simulink subsystem "petite_cana_complexeV2"  (R2024a)
settings: Solver=VariableStepAuto  StartTime=0.0  StopTime=10.0  RelTol=1e-3
undefined symbols (not defined in the file): Connection1, Connection10, Connection11, Connection12, Connection2, Connection3, Connection4, Connection5, Connection6, Connection7, Connection8, Connection9, longueur_cana, pipeline, X, Y, Z
libraries: sm_lib x27, nesl_utility x12
settings Model: Creator=vincp  LastModifiedBy=VincentPERRET

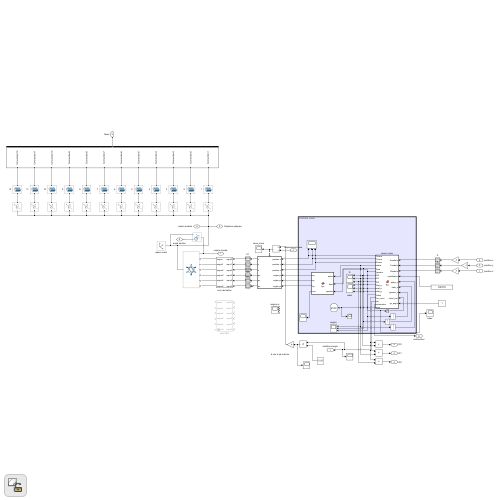
[thumbnail: Simulink's stored preview of the top-level diagram]
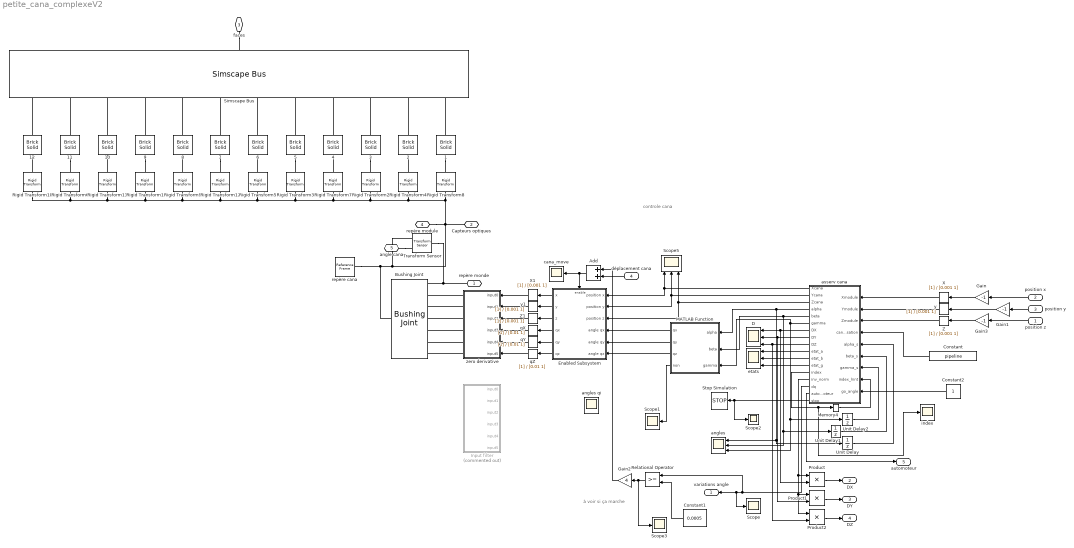
== system petite_cana_complexeV2 ==
  note: à voir si ça marche
  note: controle cana
  position z : Inport
  position x : Inport  Port=2
  position y : Inport  Port=3
  déplacement cana : Inport  Port=4
  " 1" : sm_lib/Body Elements/Brick Solid  BrickDimensions=dim_cana  BrickDimensionsUnits=m  ExportEntireGeometry=on  InertiaType=CalculateFromGeometry  BasedOnType=Mass  Density=1000  DensityUnits=kg/m^3  Mass=0  MassUnits=kg  CenterOfMass=[0 0 0]  CenterOfMassUnits=m  MomentsOfInertia=[1 1 1]  MomentsOfInertiaUnits=kg*m^2  ProductsOfInertia=[0 0 0]  ProductsOfInertiaUnits=kg*m^2  GraphicType=FromGeometry  MarkerShape=Sphere  MarkerSize=10  GraphicVisPropType=SimpleVisualProperties  GraphicDiffuseColor=[0.0 0.0 0.0]  GraphicOpacity=0.3  GraphicSpecularColor=[0.5 0.5 0.5 1.0]  GraphicAmbientColor=[0.15 0.15 0.15 1.0]  GraphicEmissiveColor=[0.0 0.0 0.0 1.0]  GraphicShininess=75  DoExposeReferenceFrame=on  SerializedFrames=<Frames/>
  " 2" : sm_lib/Body Elements/Brick Solid  BrickDimensions=dim_cana  BrickDimensionsUnits=m  ExportEntireGeometry=on  InertiaType=CalculateFromGeometry  BasedOnType=Mass  Density=1000  DensityUnits=kg/m^3  Mass=0  MassUnits=kg  CenterOfMass=[0 0 0]  CenterOfMassUnits=m  MomentsOfInertia=[1 1 1]  MomentsOfInertiaUnits=kg*m^2  ProductsOfInertia=[0 0 0]  ProductsOfInertiaUnits=kg*m^2  GraphicType=FromGeometry  MarkerShape=Sphere  MarkerSize=10  GraphicVisPropType=SimpleVisualProperties  GraphicDiffuseColor=[0.0 0.0 0.0]  GraphicOpacity=0.3  GraphicSpecularColor=[0.5 0.5 0.5 1.0]  GraphicAmbientColor=[0.15 0.15 0.15 1.0]  GraphicEmissiveColor=[0.0 0.0 0.0 1.0]  GraphicShininess=75  DoExposeReferenceFrame=on  SerializedFrames=<Frames/>
  {3,8,10,12} (4 alike) : sm_lib/Body Elements/Brick Solid  BrickDimensions=dim_cana  BrickDimensionsUnits=m  ExportEntireGeometry=on  InertiaType=CalculateFromGeometry  BasedOnType=Mass  Density=0  DensityUnits=kg/m^3  Mass=0  MassUnits=kg  CenterOfMass=[0 0 0]  CenterOfMassUnits=m  MomentsOfInertia=[1 1 1]  MomentsOfInertiaUnits=kg*m^2  ProductsOfInertia=[0 0 0]  ProductsOfInertiaUnits=kg*m^2  GraphicType=FromGeometry  MarkerShape=Sphere  MarkerSize=10  GraphicVisPropType=SimpleVisualProperties  GraphicDiffuseColor=[0.0 0.0 0.0]  GraphicOpacity=0.3  GraphicSpecularColor=[0.5 0.5 0.5 1.0]  GraphicAmbientColor=[0.15 0.15 0.15 1.0]  GraphicEmissiveColor=[0.0 0.0 0.0 1.0]  GraphicShininess=75  DoExposeReferenceFrame=on  SerializedFrames=<Frames/>
  {4..7,9,11} (6 alike) : sm_lib/Body Elements/Brick Solid  BrickDimensions=dim_cana  BrickDimensionsUnits=m  ExportEntireGeometry=on  InertiaType=CalculateFromGeometry  BasedOnType=Mass  Density=1000  DensityUnits=kg/m^3  Mass=0  MassUnits=kg  CenterOfMass=[0 0 0]  CenterOfMassUnits=m  MomentsOfInertia=[1 1 1]  MomentsOfInertiaUnits=kg*m^2  ProductsOfInertia=[0 0 0]  ProductsOfInertiaUnits=kg*m^2  GraphicType=FromGeometry  MarkerShape=Sphere  MarkerSize=10  GraphicVisPropType=SimpleVisualProperties  GraphicDiffuseColor=[0.0 0.0 0.0]  GraphicOpacity=0.3  GraphicSpecularColor=[0.5 0.5 0.5 1.0]  GraphicAmbientColor=[0.15 0.15 0.15 1.0]  GraphicEmissiveColor=[0.0 0.0 0.0 1.0]  GraphicShininess=75  DoExposeReferenceFrame=on  SerializedFrames=<Frames/>
  Add : Sum
  Bushing Joint : sm_lib/Joints/Bushing Joint  JointMode=Normal  CompositeWrenchDir=FollowerOnBase  CompositeWrenchFrame=BaseFrame  SenseConstraintForce=off  SenseConstraintTorque=off  SenseTotalForce=off  SenseTotalTorque=off  PxPositionTargetSpecify=off  PxPositionTargetPriority=High  PxPositionTargetValue=0  PxPositionTargetValueUnits=m  PxVelocityTargetSpecify=off  PxVelocityTargetPriority=High  PxVelocityTargetValue=0  PxVelocityTargetValueUnits=m/s  PxEquilibriumPosition=0  PxEquilibriumPositionUnits=m  PxSpringStiffness=0  PxSpringStiffnessUnits=N/m  PxDampingCoefficient=0  PxDampingCoefficientUnits=N/(m/s)  PxLowerLimitSpecify=off  PxLowerLimitBound=-1  PxLowerLimitBoundUnits=m  PxLowerLimitStiffness=1e6  PxLowerLimitStiffnessUnits=N/m  PxLowerLimitDamping=1e3  PxLowerLimitDampingUnits=N/(m/s)  PxLowerLimitTransitionRegionWidth=1e-4  PxLowerLimitTransitionRegionWidthUnits=m  PxUpperLimitSpecify=off  PxUpperLimitBound=1  PxUpperLimitBoundUnits=m  PxUpperLimitStiffness=1e6  PxUpperLimitStiffnessUnits=N/m  PxUpperLimitDamping=1e3  PxUpperLimitDampingUnits=N/(m/s)  PxUpperLimitTransitionRegionWidth=1e-4  PxUpperLimitTransitionRegionWidthUnits=m  PxTorqueActuationMode=ComputedTorque  PxMotionActuationMode=InputMotion  PxSensePosition=off  PxSenseVelocity=off  PxSenseAcceleration=off  PxSenseTorqueForce=off  PxSenseLowerLimitTorqueForce=off  PxSenseUpperLimitTorqueForce=off  PyPositionTargetSpecify=off  PyPositionTargetPriority=High  PyPositionTargetValue=0  PyPositionTargetValueUnits=m  PyVelocityTargetSpecify=off  PyVelocityTargetPriority=High  PyVelocityTargetValue=0  PyVelocityTargetValueUnits=m/s  PyEquilibriumPosition=0  PyEquilibriumPositionUnits=m  PySpringStiffness=0  PySpringStiffnessUnits=N/m  PyDampingCoefficient=0  PyDampingCoefficientUnits=N/(m/s)  PyLowerLimitSpecify=off  PyLowerLimitBound=-1  PyLowerLimitBoundUnits=m  PyLowerLimitStiffness=1e6  PyLowerLimitStiffnessUnits=N/m  PyLowerLimitDamping=1e3  PyLowerLimitDampingUnits=N/(m/s)  PyLowerLimitTransitionRegionWidth=1e-4  PyLowerLimitTransitionRegionWidthUnits=m  PyUpperLimitSpecify=off  PyUpperLimitBound=1  PyUpperLimitBoundUnits=m  PyUpperLimitStiffness=1e6  PyUpperLimitStiffnessUnits=N/m  PyUpperLimitDamping=1e3  PyUpperLimitDampingUnits=N/(m/s)  PyUpperLimitTransitionRegionWidth=1e-4  PyUpperLimitTransitionRegionWidthUnits=m  PyTorqueActuationMode=ComputedTorque  PyMotionActuationMode=InputMotion  PySensePosition=off  PySenseVelocity=off  PySenseAcceleration=off  PySenseTorqueForce=off  PySenseLowerLimitTorqueForce=off  PySenseUpperLimitTorqueForce=off  PzPositionTargetSpecify=off  PzPositionTargetPriority=High  PzPositionTargetValue=0  PzPositionTargetValueUnits=m  PzVelocityTargetSpecify=off  PzVelocityTargetPriority=High  PzVelocityTargetValue=0  PzVelocityTargetValueUnits=m/s  PzEquilibriumPosition=0  PzEquilibriumPositionUnits=m  PzSpringStiffness=0  PzSpringStiffnessUnits=N/m  PzDampingCoefficient=0  PzDampingCoefficientUnits=N/(m/s)  PzLowerLimitSpecify=off  PzLowerLimitBound=-1  PzLowerLimitBoundUnits=m  PzLowerLimitStiffness=1e6  PzLowerLimitStiffnessUnits=N/m  PzLowerLimitDamping=1e3  PzLowerLimitDampingUnits=N/(m/s)  PzLowerLimitTransitionRegionWidth=1e-4  PzLowerLimitTransitionRegionWidthUnits=m  PzUpperLimitSpecify=off  PzUpperLimitBound=1  PzUpperLimitBoundUnits=m  PzUpperLimitStiffness=1e6  PzUpperLimitStiffnessUnits=N/m  PzUpperLimitDamping=1e3  PzUpperLimitDampingUnits=N/(m/s)  PzUpperLimitTransitionRegionWidth=1e-4  PzUpperLimitTransitionRegionWidthUnits=m  PzTorqueActuationMode=ComputedTorque  PzMotionActuationMode=InputMotion  PzSensePosition=off  PzSenseVelocity=off  PzSenseAcceleration=off  PzSenseTorqueForce=off  PzSenseLowerLimitTorqueForce=off  PzSenseUpperLimitTorqueForce=off  RxPositionTargetSpecify=off  RxPositionTargetPriority=High  RxPositionTargetValue=0  RxPositionTargetValueUnits=deg  RxVelocityTargetSpecify=off  RxVelocityTargetPriority=High  RxVelocityTargetValue=0  RxVelocityTargetValueUnits=deg/s  RxEquilibriumPosition=0  RxEquilibriumPositionUnits=deg  RxSpringStiffness=0  RxSpringStiffnessUnits=N*m/deg  RxDampingCoefficient=0  RxDampingCoefficientUnits=N*m/(deg/s)  RxLowerLimitSpecify=off  RxLowerLimitBound=-90  RxLowerLimitBoundUnits=deg  RxLowerLimitStiffness=1e4  RxLowerLimitStiffnessUnits=N*m/deg  RxLowerLimitDamping=10  RxLowerLimitDampingUnits=N*m/(deg/s)  RxLowerLimitTransitionRegionWidth=0.1  RxLowerLimitTransitionRegionWidthUnits=deg  RxUpperLimitSpecify=off  RxUpperLimitBound=90  RxUpperLimitBoundUnits=deg  RxUpperLimitStiffness=1e4  RxUpperLimitStiffnessUnits=N*m/deg  RxUpperLimitDamping=10  RxUpperLimitDampingUnits=N*m/(deg/s)  RxUpperLimitTransitionRegionWidth=0.1  RxUpperLimitTransitionRegionWidthUnits=deg  RxTorqueActuationMode=ComputedTorque  RxMotionActuationMode=InputMotion  RxSensePosition=off  RxSenseVelocity=off  RxSenseAcceleration=off  RxSenseTorqueForce=off  RxSenseLowerLimitTorqueForce=off  RxSenseUpperLimitTorqueForce=off  RyPositionTargetSpecify=off  RyPositionTargetPriority=High  RyPositionTargetValue=0  RyPositionTargetValueUnits=deg  RyVelocityTargetSpecify=off  RyVelocityTargetPriority=High  RyVelocityTargetValue=0  RyVelocityTargetValueUnits=deg/s  RyEquilibriumPosition=0  RyEquilibriumPositionUnits=deg  RySpringStiffness=0  RySpringStiffnessUnits=N*m/deg  RyDampingCoefficient=0  RyDampingCoefficientUnits=N*m/(deg/s)  RyLowerLimitSpecify=off  RyLowerLimitBound=-90  RyLowerLimitBoundUnits=deg  RyLowerLimitStiffness=1e4  RyLowerLimitStiffnessUnits=N*m/deg  RyLowerLimitDamping=10  RyLowerLimitDampingUnits=N*m/(deg/s)  RyLowerLimitTransitionRegionWidth=0.1  RyLowerLimitTransitionRegionWidthUnits=deg  RyUpperLimitSpecify=off  RyUpperLimitBound=90  RyUpperLimitBoundUnits=deg  RyUpperLimitStiffness=1e4  RyUpperLimitStiffnessUnits=N*m/deg  RyUpperLimitDamping=10  RyUpperLimitDampingUnits=N*m/(deg/s)  RyUpperLimitTransitionRegionWidth=0.1  RyUpperLimitTransitionRegionWidthUnits=deg  RyTorqueActuationMode=ComputedTorque  RyMotionActuationMode=InputMotion  RySensePosition=off  RySenseVelocity=off  RySenseAcceleration=off  RySenseTorqueForce=off  RySenseLowerLimitTorqueForce=off  RySenseUpperLimitTorqueForce=off  RzPositionTargetSpecify=off  RzPositionTargetPriority=High  RzPositionTargetValue=0  RzPositionTargetValueUnits=deg  RzVelocityTargetSpecify=off  RzVelocityTargetPriority=High  RzVelocityTargetValue=0  RzVelocityTargetValueUnits=deg/s  RzEquilibriumPosition=0  RzEquilibriumPositionUnits=deg  RzSpringStiffness=0  RzSpringStiffnessUnits=N*m/deg  RzDampingCoefficient=0  RzDampingCoefficientUnits=N*m/(deg/s)  RzLowerLimitSpecify=off  RzLowerLimitBound=-90  RzLowerLimitBoundUnits=deg  RzLowerLimitStiffness=1e4  RzLowerLimitStiffnessUnits=N*m/deg  RzLowerLimitDamping=10  RzLowerLimitDampingUnits=N*m/(deg/s)  RzLowerLimitTransitionRegionWidth=0.1  RzLowerLimitTransitionRegionWidthUnits=deg  RzUpperLimitSpecify=off  RzUpperLimitBound=90  RzUpperLimitBoundUnits=deg  RzUpperLimitStiffness=1e4  RzUpperLimitStiffnessUnits=N*m/deg  RzUpperLimitDamping=10  RzUpperLimitDampingUnits=N*m/(deg/s)  RzUpperLimitTransitionRegionWidth=0.1  RzUpperLimitTransitionRegionWidthUnits=deg  RzTorqueActuationMode=ComputedTorque  RzMotionActuationMode=InputMotion  RzSensePosition=off  RzSenseVelocity=off  RzSenseAcceleration=off  RzSenseTorqueForce=off  RzSenseLowerLimitTorqueForce=off  RzSenseUpperLimitTorqueForce=off
  Constant : Constant  Value=pipeline
  Constant1 : Constant  Value=0.0005
  Constant2 : Constant
  D : Scope  NumInputPorts=3
  Enabled Subsystem : Subsystem  TreatAsAtomicUnit=on
  Gain : Gain  Gain=-1
  Gain1 : Gain  Gain=-1
  Gain2 : Gain  Gain=4
  Gain3 : Gain  Gain=-1
  Input filter : Subsystem  Commented=on
  MATLAB Function : MATLAB Function  TreatAsAtomicUnit=on
  Memory4 : Memory  InitialCondition=1  InheritSampleTime=on  LinearizeAsDelay=on
  Product : Product
  Product1 : Product
  Product2 : Product
  Relational Operator : RelationalOperator  OutDataTypeStr=boolean  RndMeth=Simplest  InputSameDT=off
  Rigid Transform1 : sm_lib/Frames and Transforms/Rigid Transform  RotationMethod=StandardAxis  FollAlignAxisA=+X  BaseAlignAxisA=+Y  FollAlignAxisB=+Y  BaseAlignAxisB=+Z  RotationStandardAxis=+Z  RotationAngle=-60  RotationAngleUnits=deg  RotationArbitraryAxis=[0 0 1]  RotationSequenceAxes=FollowerAxes  RotationSequence=XYX  RotationSequenceAngles=[0 0 0]  RotationSequenceAnglesUnits=deg  RotationMatrix=[1 0 0; 0 1 0; 0 0 1]  Quaternion=[1 0 0 0]  TranslationMethod=Cartesian  TranslationCartesianOffset=[-125*sin(4*pi/12) -125*cos(4*pi/12) longueur_cana*500-150]  TranslationCartesianOffsetUnits=mm  TranslationStandardAxis=+Y  TranslationStandardOffset=125  TranslationStandardOffsetUnits=mm  TranslationROffset=0  TranslationROffsetUnits=m  TranslationThetaOffset=0  TranslationThetaOffsetUnits=deg  TranslationZOffset=0  TranslationZOffsetUnits=m
  Rigid Transform10 : sm_lib/Frames and Transforms/Rigid Transform  RotationMethod=StandardAxis  FollAlignAxisA=+X  BaseAlignAxisA=+Y  FollAlignAxisB=+Y  BaseAlignAxisB=+Z  RotationStandardAxis=+Z  RotationAngle=90  RotationAngleUnits=deg  RotationArbitraryAxis=[0 0 1]  RotationSequenceAxes=FollowerAxes  RotationSequence=XYX  RotationSequenceAngles=[0 0 0]  RotationSequenceAnglesUnits=deg  RotationMatrix=[1 0 0; 0 1 0; 0 0 1]  Quaternion=[1 0 0 0]  TranslationMethod=Cartesian  TranslationCartesianOffset=[-125 0 longueur_cana*500-150]  TranslationCartesianOffsetUnits=mm  TranslationStandardAxis=+Y  TranslationStandardOffset=125  TranslationStandardOffsetUnits=mm  TranslationROffset=0  TranslationROffsetUnits=m  TranslationThetaOffset=0  TranslationThetaOffsetUnits=deg  TranslationZOffset=0  TranslationZOffsetUnits=m
  Rigid Transform11 : sm_lib/Frames and Transforms/Rigid Transform  RotationMethod=StandardAxis  FollAlignAxisA=+X  BaseAlignAxisA=+Y  FollAlignAxisB=+Y  BaseAlignAxisB=+Z  RotationStandardAxis=+Z  RotationAngle=30  RotationAngleUnits=deg  RotationArbitraryAxis=[0 0 1]  RotationSequenceAxes=FollowerAxes  RotationSequence=XYX  RotationSequenceAngles=[0 0 0]  RotationSequenceAnglesUnits=deg  RotationMatrix=[1 0 0; 0 1 0; 0 0 1]  Quaternion=[1 0 0 0]  TranslationMethod=Cartesian  TranslationCartesianOffset=[125*sin(14*pi/12) -125*cos(14*pi/12) longueur_cana*500-150]  TranslationCartesianOffsetUnits=mm  TranslationStandardAxis=+Y  TranslationStandardOffset=125  TranslationStandardOffsetUnits=mm  TranslationROffset=0  TranslationROffsetUnits=m  TranslationThetaOffset=0  TranslationThetaOffsetUnits=deg  TranslationZOffset=0  TranslationZOffsetUnits=m
  Rigid Transform12 : sm_lib/Frames and Transforms/Rigid Transform  RotationMethod=StandardAxis  FollAlignAxisA=+X  BaseAlignAxisA=+Y  FollAlignAxisB=+Y  BaseAlignAxisB=+Z  RotationStandardAxis=+Z  RotationAngle=-30  RotationAngleUnits=deg  RotationArbitraryAxis=[0 0 1]  RotationSequenceAxes=FollowerAxes  RotationSequence=XYX  RotationSequenceAngles=[0 0 0]  RotationSequenceAnglesUnits=deg  RotationMatrix=[1 0 0; 0 1 0; 0 0 1]  Quaternion=[1 0 0 0]  TranslationMethod=Cartesian  TranslationCartesianOffset=[-125*sin(2*pi/12) -125*cos(2*pi/12) longueur_cana*500-150]  TranslationCartesianOffsetUnits=mm  TranslationStandardAxis=+Y  TranslationStandardOffset=125  TranslationStandardOffsetUnits=mm  TranslationROffset=0  TranslationROffsetUnits=m  TranslationThetaOffset=0  TranslationThetaOffsetUnits=deg  TranslationZOffset=0  TranslationZOffsetUnits=m
  Rigid Transform2 : sm_lib/Frames and Transforms/Rigid Transform  RotationMethod=StandardAxis  FollAlignAxisA=+X  BaseAlignAxisA=+Y  FollAlignAxisB=+Y  BaseAlignAxisB=+Z  RotationStandardAxis=+Z  RotationAngle=60  RotationAngleUnits=deg  RotationArbitraryAxis=[0 0 1]  RotationSequenceAxes=FollowerAxes  RotationSequence=XYX  RotationSequenceAngles=[0 0 0]  RotationSequenceAnglesUnits=deg  RotationMatrix=[1 0 0; 0 1 0; 0 0 1]  Quaternion=[1 0 0 0]  TranslationMethod=Cartesian  TranslationCartesianOffset=[125*sin(4*pi/12) -125*cos(4*pi/12) longueur_cana*500-150]  TranslationCartesianOffsetUnits=mm  TranslationStandardAxis=+Y  TranslationStandardOffset=125  TranslationStandardOffsetUnits=mm  TranslationROffset=0  TranslationROffsetUnits=m  TranslationThetaOffset=0  TranslationThetaOffsetUnits=deg  TranslationZOffset=0  TranslationZOffsetUnits=m
  Rigid Transform3 : sm_lib/Frames and Transforms/Rigid Transform  RotationMethod=StandardAxis  FollAlignAxisA=+X  BaseAlignAxisA=+Y  FollAlignAxisB=+Y  BaseAlignAxisB=+Z  RotationStandardAxis=+Z  RotationAngle=120  RotationAngleUnits=deg  RotationArbitraryAxis=[0 0 1]  RotationSequenceAxes=FollowerAxes  RotationSequence=XYX  RotationSequenceAngles=[0 0 0]  RotationSequenceAnglesUnits=deg  RotationMatrix=[1 0 0; 0 1 0; 0 0 1]  Quaternion=[1 0 0 0]  TranslationMethod=Cartesian  TranslationCartesianOffset=[125*sin(8*pi/12) -125*cos(8*pi/12) longueur_cana*500-150]  TranslationCartesianOffsetUnits=mm  TranslationStandardAxis=+Y  TranslationStandardOffset=125  TranslationStandardOffsetUnits=mm  TranslationROffset=0  TranslationROffsetUnits=m  TranslationThetaOffset=0  TranslationThetaOffsetUnits=deg  TranslationZOffset=0  TranslationZOffsetUnits=m
  Rigid Transform4 : sm_lib/Frames and Transforms/Rigid Transform  RotationMethod=StandardAxis  FollAlignAxisA=+X  BaseAlignAxisA=+Y  FollAlignAxisB=+Y  BaseAlignAxisB=+Z  RotationStandardAxis=+Z  RotationAngle=30  RotationAngleUnits=deg  RotationArbitraryAxis=[0 0 1]  RotationSequenceAxes=FollowerAxes  RotationSequence=XYX  RotationSequenceAngles=[0 0 0]  RotationSequenceAnglesUnits=deg  RotationMatrix=[1 0 0; 0 1 0; 0 0 1]  Quaternion=[1 0 0 0]  TranslationMethod=Cartesian  TranslationCartesianOffset=[125*sin(2*pi/12) -125*cos(2*pi/12) longueur_cana*500-150]  TranslationCartesianOffsetUnits=mm  TranslationStandardAxis=+Y  TranslationStandardOffset=125  TranslationStandardOffsetUnits=mm  TranslationROffset=0  TranslationROffsetUnits=m  TranslationThetaOffset=0  TranslationThetaOffsetUnits=deg  TranslationZOffset=0  TranslationZOffsetUnits=m
  Rigid Transform5 : sm_lib/Frames and Transforms/Rigid Transform  RotationMethod=StandardAxis  FollAlignAxisA=+X  BaseAlignAxisA=+Y  FollAlignAxisB=+Y  BaseAlignAxisB=+Z  RotationStandardAxis=+Z  RotationAngle=150  RotationAngleUnits=deg  RotationArbitraryAxis=[0 0 1]  RotationSequenceAxes=FollowerAxes  RotationSequence=XYX  RotationSequenceAngles=[0 0 0]  RotationSequenceAnglesUnits=deg  RotationMatrix=[1 0 0; 0 1 0; 0 0 1]  Quaternion=[1 0 0 0]  TranslationMethod=Cartesian  TranslationCartesianOffset=[125*sin(10*pi/12) -125*cos(10*pi/12) longueur_cana*500-150]  TranslationCartesianOffsetUnits=mm  TranslationStandardAxis=+Y  TranslationStandardOffset=125  TranslationStandardOffsetUnits=mm  TranslationROffset=0  TranslationROffsetUnits=m  TranslationThetaOffset=0  TranslationThetaOffsetUnits=deg  TranslationZOffset=0  TranslationZOffsetUnits=m
  Rigid Transform6 : sm_lib/Frames and Transforms/Rigid Transform  RotationMethod=StandardAxis  FollAlignAxisA=+X  BaseAlignAxisA=+Y  FollAlignAxisB=+Y  BaseAlignAxisB=+Z  RotationStandardAxis=+Z  RotationAngle=60  RotationAngleUnits=deg  RotationArbitraryAxis=[0 0 1]  RotationSequenceAxes=FollowerAxes  RotationSequence=XYX  RotationSequenceAngles=[0 0 0]  RotationSequenceAnglesUnits=deg  RotationMatrix=[1 0 0; 0 1 0; 0 0 1]  Quaternion=[1 0 0 0]  TranslationMethod=Cartesian  TranslationCartesianOffset=[-125*cos(pi/6) 125*sin(pi/6) longueur_cana*500-150]  TranslationCartesianOffsetUnits=mm  TranslationStandardAxis=+Y  TranslationStandardOffset=125  TranslationStandardOffsetUnits=mm  TranslationROffset=0  TranslationROffsetUnits=m  TranslationThetaOffset=0  TranslationThetaOffsetUnits=deg  TranslationZOffset=0  TranslationZOffsetUnits=m
  Rigid Transform7 : sm_lib/Frames and Transforms/Rigid Transform  RotationMethod=StandardAxis  FollAlignAxisA=+X  BaseAlignAxisA=+Y  FollAlignAxisB=+Y  BaseAlignAxisB=+Z  RotationStandardAxis=+Z  RotationAngle=90  RotationAngleUnits=deg  RotationArbitraryAxis=[0 0 1]  RotationSequenceAxes=FollowerAxes  RotationSequence=XYX  RotationSequenceAngles=[0 0 0]  RotationSequenceAnglesUnits=deg  RotationMatrix=[1 0 0; 0 1 0; 0 0 1]  Quaternion=[1 0 0 0]  TranslationMethod=Cartesian  TranslationCartesianOffset=[125 0 longueur_cana*500-150]  TranslationCartesianOffsetUnits=mm  TranslationStandardAxis=+Y  TranslationStandardOffset=125  TranslationStandardOffsetUnits=mm  TranslationROffset=0  TranslationROffsetUnits=m  TranslationThetaOffset=0  TranslationThetaOffsetUnits=deg  TranslationZOffset=0  TranslationZOffsetUnits=m
  Rigid Transform8 : sm_lib/Frames and Transforms/Rigid Transform  RotationMethod=StandardAxis  FollAlignAxisA=+X  BaseAlignAxisA=+Y  FollAlignAxisB=+Y  BaseAlignAxisB=+Z  RotationStandardAxis=+Z  RotationAngle=0  RotationAngleUnits=deg  RotationArbitraryAxis=[0 0 1]  RotationSequenceAxes=FollowerAxes  RotationSequence=XYX  RotationSequenceAngles=[0 0 0]  RotationSequenceAnglesUnits=deg  RotationMatrix=[1 0 0; 0 1 0; 0 0 1]  Quaternion=[1 0 0 0]  TranslationMethod=Cartesian  TranslationCartesianOffset=[0 -125 longueur_cana*500-150]  TranslationCartesianOffsetUnits=mm  TranslationStandardAxis=+Y  TranslationStandardOffset=125  TranslationStandardOffsetUnits=mm  TranslationROffset=0  TranslationROffsetUnits=m  TranslationThetaOffset=0  TranslationThetaOffsetUnits=deg  TranslationZOffset=0  TranslationZOffsetUnits=m
  Rigid Transform9 : sm_lib/Frames and Transforms/Rigid Transform  RotationMethod=StandardAxis  FollAlignAxisA=+X  BaseAlignAxisA=+Y  FollAlignAxisB=+Y  BaseAlignAxisB=+Z  RotationStandardAxis=+Z  RotationAngle=0  RotationAngleUnits=deg  RotationArbitraryAxis=[0 0 1]  RotationSequenceAxes=FollowerAxes  RotationSequence=XYX  RotationSequenceAngles=[0 0 0]  RotationSequenceAnglesUnits=deg  RotationMatrix=[1 0 0; 0 1 0; 0 0 1]  Quaternion=[1 0 0 0]  TranslationMethod=Cartesian  TranslationCartesianOffset=[0 125 longueur_cana*500-150]  TranslationCartesianOffsetUnits=mm  TranslationStandardAxis=+Y  TranslationStandardOffset=125  TranslationStandardOffsetUnits=mm  TranslationROffset=0  TranslationROffsetUnits=m  TranslationThetaOffset=0  TranslationThetaOffsetUnits=deg  TranslationZOffset=0  TranslationZOffsetUnits=m
  Scope{,1..3} (4 alike) : Scope
  Scope5 : Scope  NumInputPorts=3
  Simscape Bus : SimscapeBus  HierarchyStrings=Connection12;Connection11;Connection10;Connection9;Connection8;Connection7;Connection6;Connection5;Connection4;Connection3;Connection2;Connection1
  Stop Simulation : Stop
  Transform Sensor : sm_lib/Frames and Transforms/Transform Sensor  MeasurementFrame=World  RotationSequence=XYX  SenseAngle=on  SenseAxis=off  SenseQ=off  SenseR=off  SenseRotationSequence=off  SenseOmegaX=off  SenseOmegaY=off  SenseOmegaZ=off  SenseOmega=off  SenseQDot=off  SenseRDot=off  SenseRotationSequenceDot=off  SenseAlphaX=off  SenseAlphaY=off  SenseAlphaZ=off  SenseAlpha=off  SenseQDDot=off  SenseRDDot=off  SenseX=off  SenseY=off  SenseZ=off  SenseXYZ=off  SenseRad=off  SenseAzim=off  SenseDist=off  SenseInc=off  SenseXDot=off  SenseYDot=off  SenseZDot=off  SenseXYZDot=off  SenseRadDot=off  SenseAzimDot=off  SenseDistDot=off  SenseIncDot=off  SenseXDDot=off  SenseYDDot=off  SenseZDDot=off  SenseXYZDDot=off  SenseRadDDot=off  SenseAzimDDot=off  SenseDistDDot=off  SenseIncDDot=off
  Unit Delay : UnitDelay  SampleTime=-1  HasFrameUpgradeWarning=on
  Unit Delay1 : UnitDelay  SampleTime=-1  HasFrameUpgradeWarning=on
  Unit Delay2 : UnitDelay  SampleTime=-1  HasFrameUpgradeWarning=on
  X : TransferFcn  Denominator=[0.001 1]
  X1 : TransferFcn  Denominator=[0.001 1]
  Z : TransferFcn  Denominator=[0.001 1]
  Z1 : TransferFcn  Denominator=[0.001 1]
  angles : Scope  NumInputPorts=3
  angles qi : Scope  NumInputPorts=3
  asserv cana : MATLAB Function  TreatAsAtomicUnit=on
  cana_move : Scope
  etats : Scope  NumInputPorts=3
  index : Scope
  qX : TransferFcn  Denominator=[0.01 1]
  qY : TransferFcn  Denominator=[0.01 1]
  qZ : TransferFcn  Denominator=[0.01 1]
  repère cana : sm_lib/Frames and Transforms/Reference Frame
  y : TransferFcn  Denominator=[0.001 1]
  y1 : TransferFcn  Denominator=[0.001 1]
  zero derivative : Subsystem
  repère monde : PMIOPort  Side=Right
  Capteurs optiques : PMIOPort  Port=2  Side=Left
  faces : PMIOPort  Port=3  Side=Left
  repère module : PMIOPort  Port=4  Side=Left
  angle cana : PMIOPort  Port=5  Side=Left
  variations angle : Outport
  DX : Outport  Port=2
  DY : Outport  Port=3
  DZ : Outport  Port=4
  automoteur : Outport  Port=5
  wires:
  position y/1 -> Gain1/1
  position z/1 -> Gain3/1
  Gain1/1 -> y/1
  Gain3/1 -> Z/1
  Gain/1 -> X/1
  asserv cana/1(Xcana) -> Scope5/1, Enabled Subsystem/1(position x)
  asserv cana/2(Ycana) -> Scope5/2, Enabled Subsystem/2(position y)
  asserv cana/3(Zcana) -> Scope5/3, Enabled Subsystem/3(position z)
  Z/1 -> asserv cana/3(Zmodule)
  asserv cana/7(DX) -> D/1, Product/2
  asserv cana/9(DZ) -> D/3, Product2/2
  Constant/1 -> asserv cana/4(canalisation)
  asserv cana/12(etat_g) -> etats/3
  Constant2/1 -> asserv cana/9(go_angle)
  Memory4/1 -> asserv cana/8(index_hint)
  asserv cana/13(index) -> Memory4/1, index/1
  Unit Delay1/1 -> asserv cana/6(beta_s)
  MATLAB Function/4(non) -> Scope1/1
  y/1 -> asserv cana/2(Ymodule)
  X/1 -> asserv cana/1(Xmodule)
  asserv cana/8(DY) -> Product1/2, D/2
  Unit Delay2/1 -> asserv cana/7(gamma_s)
  Unit Delay/1 -> asserv cana/5(alpha_s)
  asserv cana/4(alpha) -> MATLAB Function/1(alpha), angles/1, Unit Delay/1
  asserv cana/5(beta) -> MATLAB Function/2(beta), angles/2, Unit Delay1/1
  Product/1 -> DX/1
  Product1/1 -> DY/1
  asserv cana/14(inv_norm) -> Product/1, Product1/1, Product2/1
  Product2/1 -> DZ/1
  asserv cana/15(dq) -> Scope/1, variations angle/1, Relational Operator/1
  asserv cana/16(automoteur) -> automoteur/1
  Enabled Subsystem/1(x) -> X1/1
  Enabled Subsystem/2(y) -> y1/1
  Enabled Subsystem/3(z) -> Z1/1
  Enabled Subsystem/4(qx) -> qX/1
  Enabled Subsystem/5(qy) -> qY/1
  Enabled Subsystem/6(qz) -> qZ/1
  X1/1 -> zero derivative/1(input0)
  y1/1 -> zero derivative/2(input1)
  Z1/1 -> zero derivative/3(input2)
  position x/1 -> Gain/1
  Add/1 -> cana_move/1, Enabled Subsystem/Enable
  asserv cana/6(gamma) -> MATLAB Function/3(gamma), angles/3, Unit Delay2/1
  MATLAB Function/1(qx) -> Enabled Subsystem/4(angle qx)
  MATLAB Function/2(qy) -> Enabled Subsystem/5(angle qy)
  asserv cana/17(stop) -> Stop Simulation/1, Scope2/1
  Constant1/1 -> Relational Operator/2
  Relational Operator/1 -> Scope3/1, Gain2/1
  Gain2/1 -> Add/1
  déplacement cana/1 -> Add/2
  asserv cana/10(etat_a) -> etats/1
  asserv cana/11(etat_b) -> etats/2
  MATLAB Function/3(qz) -> Enabled Subsystem/6(angle qz)
  qX/1 -> zero derivative/4(input3)
  qY/1 -> zero derivative/5(input4)
  qZ/1 -> zero derivative/6(input5)
  connections:
  Rigid Transform10/LConn1 -- repère module/RConn1 -- Capteurs optiques/RConn1 -- Bushing Joint/RConn1 -- repère cana/RConn1 -- Transform Sensor/RConn1 -- Rigid Transform8/LConn1 -- Rigid Transform4/LConn1 -- Rigid Transform2/LConn1 -- Rigid Transform7/LConn1 -- Rigid Transform3/LConn1 -- Rigid Transform5/LConn1 -- Rigid Transform12/LConn1 -- Rigid Transform9/LConn1 -- Rigid Transform1/LConn1 -- Rigid Transform11/LConn1 -- Rigid Transform6/LConn1
  Transform Sensor/LConn1 -- repère monde/RConn1 -- Bushing Joint/LConn1
  " 1"/RConn1 -- Rigid Transform8/RConn1
  " 1"/LConn1 -- Simscape Bus/LConn12
  6/LConn1 -- Simscape Bus/LConn7
  3/RConn1 -- Rigid Transform2/RConn1
  5/LConn1 -- Simscape Bus/LConn8
  3/LConn1 -- Simscape Bus/LConn10
  " 2"/LConn1 -- Simscape Bus/LConn11
  faces/RConn1 -- Simscape Bus/RConn1
  Rigid Transform11/RConn1 -- 10/RConn1
  11/LConn1 -- Simscape Bus/LConn2
  8/LConn1 -- Simscape Bus/LConn5
  10/LConn1 -- Simscape Bus/LConn3
  7/LConn1 -- Simscape Bus/LConn6
  12/LConn1 -- Simscape Bus/LConn1
  Rigid Transform10/RConn1 -- 12/RConn1
  11/RConn1 -- Rigid Transform6/RConn1
  7/RConn1 -- Rigid Transform12/RConn1
  Rigid Transform9/RConn1 -- 8/RConn1
  9/LConn1 -- Simscape Bus/LConn4
  9/RConn1 -- Rigid Transform1/RConn1
  Rigid Transform5/RConn1 -- 6/RConn1
  Rigid Transform4/RConn1 -- " 2"/RConn1
  5/RConn1 -- Rigid Transform3/RConn1
  Rigid Transform7/RConn1 -- 4/RConn1
  4/LConn1 -- Simscape Bus/LConn9
  zero derivative/RConn1 -- Bushing Joint/LConn2
  zero derivative/RConn2 -- Bushing Joint/LConn3
  zero derivative/RConn3 -- Bushing Joint/LConn4
  zero derivative/RConn4 -- Bushing Joint/LConn5
  zero derivative/RConn5 -- Bushing Joint/LConn6
  zero derivative/RConn6 -- Bushing Joint/LConn7
  angle cana/RConn1 -- Transform Sensor/RConn2

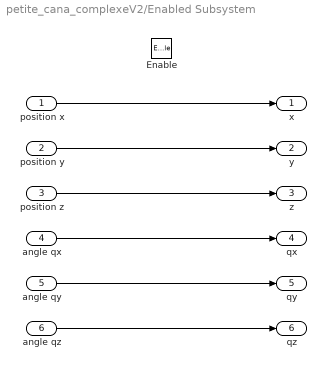
== system petite_cana_complexeV2/Enabled Subsystem ==
  position x : Inport
  position y : Inport  Port=2
  position z : Inport  Port=3
  angle qx : Inport  Port=4
  angle qy : Inport  Port=5
  angle qz : Inport  Port=6
  Enable : EnablePort
  x : Outport
  y : Outport  Port=2
  z : Outport  Port=3
  qx : Outport  Port=4
  qy : Outport  Port=5
  qz : Outport  Port=6
  wires:
  angle qz/1 -> qz/1
  angle qy/1 -> qy/1
  angle qx/1 -> qx/1
  position z/1 -> z/1
  position y/1 -> y/1
  position x/1 -> x/1

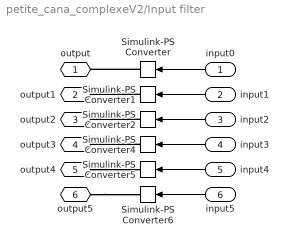
== system petite_cana_complexeV2/Input filter ==
  input0 : Inport
  input1 : Inport  Port=2
  input2 : Inport  Port=3
  input3 : Inport  Port=4
  input4 : Inport  Port=5
  input5 : Inport  Port=6
  Simulink-PS Converter : nesl_utility/Simulink-PS Converter  PhysicalDomain=network_engine_domain  SubClassName=ps_input  LeftPortType=input  RightPortType=output  PseudoPeriodic=off  Frequencies=[]  NoiseDistribution=none  NoiseParameters=[]  Unit=1  AffineConversion=off  FilteringAndDerivatives=filter  SimscapeFilterOrder=2  InputFilterTimeConstant=0.01  UdotUserProvided=0
  Simulink-PS Converter1 : nesl_utility/Simulink-PS Converter  PhysicalDomain=network_engine_domain  SubClassName=ps_input  LeftPortType=input  RightPortType=output  PseudoPeriodic=off  Frequencies=[]  NoiseDistribution=none  NoiseParameters=[]  Unit=1  AffineConversion=off  FilteringAndDerivatives=filter  SimscapeFilterOrder=2  InputFilterTimeConstant=0.01  UdotUserProvided=0
  Simulink-PS Converter2 : nesl_utility/Simulink-PS Converter  PhysicalDomain=network_engine_domain  SubClassName=ps_input  LeftPortType=input  RightPortType=output  PseudoPeriodic=off  Frequencies=[]  NoiseDistribution=none  NoiseParameters=[]  Unit=1  AffineConversion=off  FilteringAndDerivatives=filter  SimscapeFilterOrder=2  InputFilterTimeConstant=0.01  UdotUserProvided=0
  Simulink-PS Converter4 : nesl_utility/Simulink-PS Converter  PhysicalDomain=network_engine_domain  SubClassName=ps_input  LeftPortType=input  RightPortType=output  PseudoPeriodic=off  Frequencies=[]  NoiseDistribution=none  NoiseParameters=[]  Unit=1  AffineConversion=off  FilteringAndDerivatives=filter  SimscapeFilterOrder=2  InputFilterTimeConstant=0.1  UdotUserProvided=0
  Simulink-PS Converter5 : nesl_utility/Simulink-PS Converter  PhysicalDomain=network_engine_domain  SubClassName=ps_input  LeftPortType=input  RightPortType=output  PseudoPeriodic=off  Frequencies=[]  NoiseDistribution=none  NoiseParameters=[]  Unit=1  AffineConversion=off  FilteringAndDerivatives=filter  SimscapeFilterOrder=2  InputFilterTimeConstant=0.1  UdotUserProvided=0
  Simulink-PS Converter6 : nesl_utility/Simulink-PS Converter  PhysicalDomain=network_engine_domain  SubClassName=ps_input  LeftPortType=input  RightPortType=output  PseudoPeriodic=off  Frequencies=[]  NoiseDistribution=none  NoiseParameters=[]  Unit=1  AffineConversion=off  FilteringAndDerivatives=filter  SimscapeFilterOrder=2  InputFilterTimeConstant=0.1  UdotUserProvided=0
  output : PMIOPort  Side=Right
  output1 : PMIOPort  Port=2  Side=Right
  output2 : PMIOPort  Port=3  Side=Right
  output3 : PMIOPort  Port=4  Side=Right
  output4 : PMIOPort  Port=5  Side=Right
  output5 : PMIOPort  Port=6  Side=Right
  wires:
  input5/1 -> Simulink-PS Converter6/1
  input4/1 -> Simulink-PS Converter5/1
  input2/1 -> Simulink-PS Converter2/1
  input1/1 -> Simulink-PS Converter1/1
  input3/1 -> Simulink-PS Converter4/1
  input0/1 -> Simulink-PS Converter/1
  connections:
  Simulink-PS Converter1/RConn1 -- output1/RConn1
  Simulink-PS Converter2/RConn1 -- output2/RConn1
  Simulink-PS Converter4/RConn1 -- output3/RConn1
  output4/RConn1 -- Simulink-PS Converter5/RConn1
  Simulink-PS Converter/RConn1 -- output/RConn1
  output5/RConn1 -- Simulink-PS Converter6/RConn1

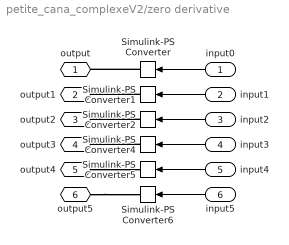
== system petite_cana_complexeV2/zero derivative ==
  input0 : Inport
  input1 : Inport  Port=2
  input2 : Inport  Port=3
  input3 : Inport  Port=4
  input4 : Inport  Port=5
  input5 : Inport  Port=6
  Simulink-PS Converter{,1..2,4..6} (6 alike) : nesl_utility/Simulink-PS Converter  PhysicalDomain=network_engine_domain  SubClassName=ps_input  LeftPortType=input  RightPortType=output  PseudoPeriodic=off  Frequencies=[]  NoiseDistribution=none  NoiseParameters=[]  Unit=1  AffineConversion=off  FilteringAndDerivatives=zero  SimscapeFilterOrder=2  InputFilterTimeConstant=0.01  UdotUserProvided=0
  output : PMIOPort  Side=Right
  output1 : PMIOPort  Port=2  Side=Right
  output2 : PMIOPort  Port=3  Side=Right
  output3 : PMIOPort  Port=4  Side=Right
  output4 : PMIOPort  Port=5  Side=Right
  output5 : PMIOPort  Port=6  Side=Right
  wires:
  input5/1 -> Simulink-PS Converter6/1
  input4/1 -> Simulink-PS Converter5/1
  input2/1 -> Simulink-PS Converter2/1
  input1/1 -> Simulink-PS Converter1/1
  input3/1 -> Simulink-PS Converter4/1
  input0/1 -> Simulink-PS Converter/1
  connections:
  Simulink-PS Converter1/RConn1 -- output1/RConn1
  Simulink-PS Converter2/RConn1 -- output2/RConn1
  Simulink-PS Converter4/RConn1 -- output3/RConn1
  output4/RConn1 -- Simulink-PS Converter5/RConn1
  Simulink-PS Converter/RConn1 -- output/RConn1
  output5/RConn1 -- Simulink-PS Converter6/RConn1

== matlab function petite_cana_complexeV2/MATLAB Function ==
  data: alpha input; beta input; qx output; gamma input; qy output; qz output; non output
function [qx,qy,qz,non] = fcn(alpha, beta, gamma)

if alpha >=pi/2 -0.05
    qy=gamma;
    qx=alpha ;
    qz=0 ;
    non=2;

elseif alpha <=-pi/2+0.05 && abs(gamma)>0.01 
    qy=pi-abs(gamma);
    qx=alpha ;
    qz=0 ;
    non=3;
    pause(0.5);
elseif abs(beta)>pi/2-0.01 && abs(gamma) >0.01
    qx=-pi/2;
    qy=pi-gamma;
    qz=0 ;
    non =1;

  
else 
    qy=beta ;
    qx=alpha ;
    qz=0 ; 
    non=0;
  
end 

end

== matlab function petite_cana_complexeV2/asserv cana ==
  data: Xmodule input; Ymodule input; Xcana output; Ycana output; Zcana output; alpha output; beta output; gamma output; Zmodule input; canalisation input; alpha_s input; beta_s input; gamma_s input; index_hint input; DX output; DY output; DZ output; etat_a output; etat_b output; etat_g output; go_angle input; index output; inv_norm output; dq output; automoteur output; stop output
function [Xcana,Ycana,Zcana,alpha,beta,gamma,DX,DY ,DZ,etat_a,etat_b, etat_g, index,inv_norm,dq,automoteur,stop] = fcn(Xmodule,Ymodule,Zmodule, canalisation,alpha_s,beta_s,gamma_s, index_hint, go_angle)
centre_module = [Xmodule Ymodule Zmodule];
pipeline=canalisation;
%distances = sqrt(sum((L_moy - centre_module).^2, 1));
% Trouver l'indice du point le plus proche
%[~, closestPointIndex] = min(distances);
% Récupérer les coordonnées du point le plus proche
%if closestPointIndex <= 1
%    closestPointIndex=closestPointIndex+1;
%end 
%closestPoint =L_moy(:, closestPointIndex);
%closest_closestPoint =L_moy(:, closestPointIndex-1);
%DX = closestPoint(1)-closest_closestPoint(1);
%DY = closestPoint(2)-closest_closestPoint(2);
%DZ = closestPoint(3)-closest_closestPoint(3);
%if DZ<=1e-4 && DZ>=-1e-4
%    DZ=0;
%end
%if DY<=1e-4 && DY>=-1e-4
%    DY=0;
%end
%if DX<=1e-4 && DX>=-1e-4
%    DX=0;
%end


if go_angle
    % Trouver l'element de cana correspondant au point
[index,stop] = findPipeIndex(centre_module, pipeline, index_hint);
tangent = findPipeTangent(centre_module, pipeline(index, :));
clipped_point = clipPointToPipe(centre_module, pipeline(index, :));

nextType =  nextPipe(pipeline,index); %Type de la cana d'après, si c'est un coude = true ou une ligne droite = false 
Type= nextPipe(pipeline,index-1) ; %Type de la cana actuelle
if nextType 
    nextEnterPoint=enterPoint(index+1,pipeline);
    distanceNextPipe= sqrt((Xmodule-nextEnterPoint(1))^2 + (Ymodule-nextEnterPoint(2))^2 + (Zmodule-nextEnterPoint(3))^2);
      
 
    if distanceNextPipe <=0.5
        automoteur = true;
    else 
        automoteur = false ;

    end 
else 
    automoteur = false ;

end

Xcana= clipped_point(1);
Ycana = clipped_point(2);
Zcana = clipped_point(3);

DX = tangent(1);
DY = tangent(2);
DZ = tangent(3);
norm_=sqrt(DX^2+DY^2+DZ^2);
if norm_ ~= 0
    inv_norm=1/norm_;
else 
    inv_norm =0;
end

% DX=0;
% DY=0;
% DZ=0;

    %Rotation autour de x :
    if abs(DZ) ==0|| abs(DY) ==0
        alpha= alpha_s;
        etat_a=0;
        deltaAngle_qx=0;
    else

        etat_a=1;
        % Calculer l'angle actuel avec atan2
        currentAngle_qx = -atan2(DY,DZ);
    
        % Différence entre l'angle actuel et l'angle précédent
        deltaAngle_qx = currentAngle_qx - alpha_s;
    
        % Gérer le cas où l'angle change de signe au-delà de π ou -π
        if deltaAngle_qx > pi
            deltaAngle_qx = deltaAngle_qx - 2*pi;
            etat_a=2;
        elseif deltaAngle_qx < -pi
            deltaAngle_qx = deltaAngle_qx + 2*pi;
            etat_a = 3;
        end
    
        % Mettre à jour l'angle accumulé    
        % if abs(deltaAngle_qx) <0.01 && Type
        %      alpha= alpha_s;
        % else
           alpha = alpha_s + deltaAngle_qx;
           % alpha = 0;
        % end

    end



    %rotation autour de y :
    if  DX==0 || abs(DZ) ==0
        beta= beta_s;
        etat_b=0;
        deltaAngle_qy=0;
    else

        etat_b=1;
        % Calculer l'angle actuel avec atan2
        currentAngle_qy = atan2(DX,sqrt(DZ^2 + DY^2)); % modif
    
        % Différence entre l'angle actuel et l'angle précédent
        deltaAngle_qy = currentAngle_qy - beta_s;
    
        % Gérer le cas où l'angle change de signe au-delà de π ou -π
        if deltaAngle_qy > pi
            deltaAngle_qy = deltaAngle_qy + 2*pi;
            etat_b=2;
        elseif deltaAngle_qy < -pi
            deltaAngle_qy = deltaAngle_qy - 2*pi;
            etat_b = 3;
        end
    
    % Mettre à jour l'angle accumulé    
        % if abs(deltaAngle_qy)  <0.01 && Type
        %      beta= beta_s;
        % else
             beta = beta_s + deltaAngle_qy;
        % end
       

    end


    % rotation autour de z :
    if  abs(DX) ==0 ||  abs(DY)==0
        gamma= gamma_s;
        etat_g=0;
        deltaAngle_qz=0;
    else

        etat_g=1;
        % Calculer l'angle actuel avec atan2
        currentAngle_qz = -atan2(-DX,-DY);
    
        % Différence entre l'angle actuel et l'angle précédent
        deltaAngle_qz = currentAngle_qz - gamma_s;
    
        % Gérer le cas où l'angle change de signe au-delà de π ou -π
        if deltaAngle_qz > pi
            deltaAngle_qz = deltaAngle_qz + 2*pi;
            etat_g=2;
        elseif deltaAngle_qz < -pi
            deltaAngle_qz = deltaAngle_qz - 2*pi;
            etat_g = 3;
        end
    
    % Mettre à jour l'angle accumulé 
        % if abs(deltaAngle_qz) <0.01 && Type
        %      gamma= gamma_s ;
        % else
            gamma = gamma_s+ deltaAngle_qz;
        % end
    end
    dq=sqrt(deltaAngle_qx^2+deltaAngle_qy^2+deltaAngle_qz^2);
else 
    alpha = 0 ;
    beta  = 0 ;
    gamma = 0 ;
    etat_a = 0;
    etat_b = 0;
    etat_g = 0;
    Xcana= 0;
    Ycana = 0;
    Zcana = 0;
    index = 1;
    DX=0;
    DY=0;
    DZ=0;
    inv_norm=1;
    dq=0;
    automoteur = false ; 
    stop = false ;
 
end

end
